simulink model "integracion_control_trayectoria"  (R2023b)
settings: Solver=FixedStepDiscrete  StartTime=0.0  StopTime=inf  RelTol=1e-3  EnableMultiTasking=on
undefined symbols (not defined in the file): LF
libraries: instrumentseriallib x3, svdutilitieslib x1, dspnetwork x1
settings Model: SimulationMode=accelerator  Creator=gianm  LastModifiedBy=gianm
settings DebuggingCC: ParameterPrecisionLossMsg=none

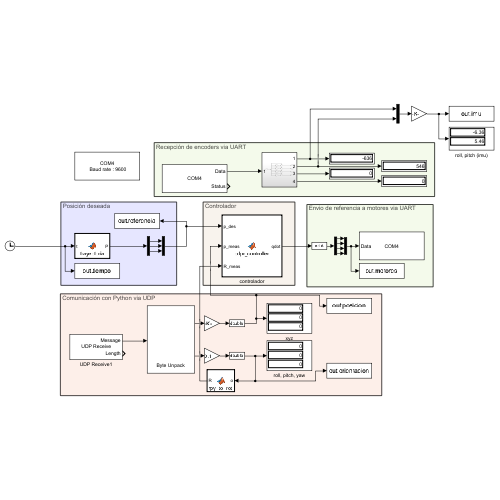
[thumbnail: Simulink's stored preview of the top-level diagram]
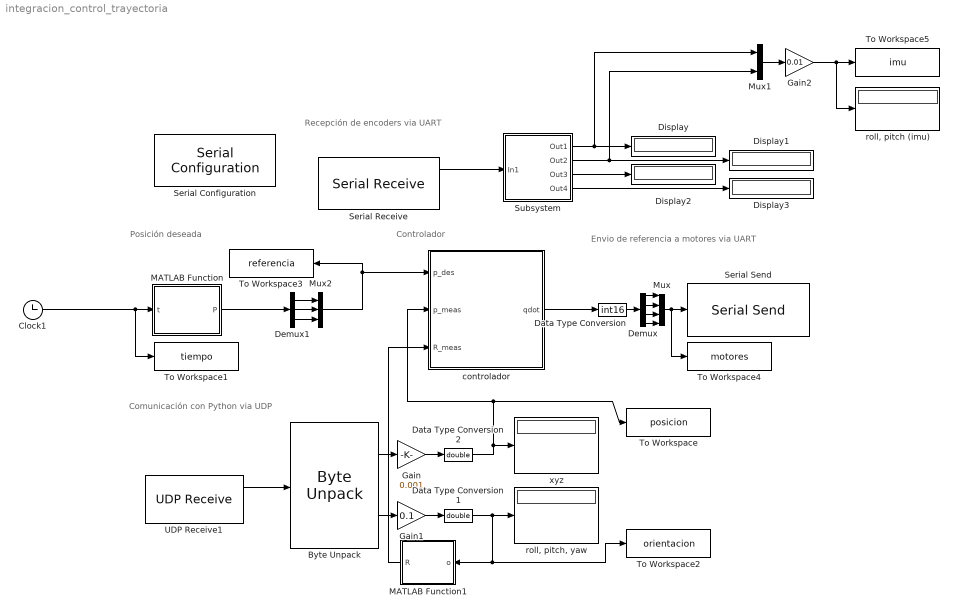
== system integracion_control_trayectoria ==
  note: Recepción de encoders via UART
  note: Controlador
  note: Envio de referencia a motores via UART
  note: Posición deseada
  note: Comunicación con Python via UDP
  Byte Unpack : svdutilitieslib/Byte Unpack  dimensions={[3,1], [3,1]}  datatypes={'int16', 'int16'}  byteAlign=1  blockPlatform=arduinoert
  Clock1 : Clock
  Data Type Conversion : DataTypeConversion  OutDataTypeStr=int16  SaturateOnIntegerOverflow=off  RndMeth=Floor
  Data Type Conversion1 : DataTypeConversion  OutDataTypeStr=double  SaturateOnIntegerOverflow=off  RndMeth=Floor
  Data Type Conversion2 : DataTypeConversion  OutDataTypeStr=double  SaturateOnIntegerOverflow=off  RndMeth=Floor
  Demux : Demux
  Demux1 : Demux  Outputs=3
  Display{,1..3} (4 alike) : Display
      settings: Format=decimal (Stored Integer)
  Gain : Gain  Gain=0.001
  Gain1 : Gain  Gain=0.1
  Gain2 : Gain  Gain=0.01
  MATLAB Function : MATLAB Function  TreatAsAtomicUnit=on
  MATLAB Function1 : MATLAB Function  TreatAsAtomicUnit=on
  Mux : Mux
  Mux1 : Mux  Inputs=2
  Mux2 : Mux  Inputs=3
  Serial Configuration : instrumentseriallib/Serial Configuration  Priority=-200000  PortSel=COM4  Port=COM4  ComPort=COM4  BaudRate=9600  DataBits=8  Parity=none  StopBits=1  ByteOrder=little-endian  FlowControl=none  Timeout=20  SimulateUsing=Interpreted execution  BlockInModel=on  aMode=1
  Serial Receive : instrumentseriallib/Serial Receive  Priority=1  PortSel=COM4  Port=COM4  ComPort=COM4  DataType=uint8  SaveDataType=uint8  ToggleHeader=on  Header=[82]  DataSize=8  ToggleTerminator=on  Terminator=LF ('\n')  CustomTerminator=[]  InputFormat=Column major  ToggleDataSize=on  EnableBlockingMode=off  ActionDataUnavailable=Output last received value  ActionWhenDataUnavailable=Output last received value  CustomValue=0  SampleTime=0.02  SimulateUsing=Interpreted execution  BlockInModel=on  aMode=1
  Serial Send : instrumentseriallib/Serial Send  Priority=1  PortSel=COM4  Port=COM4  ComPort=COM4  Header=[72]  Terminator=LF ('\n')  CustomTerminator=[]  EnableBlockingMode=off  SimulateUsing=Interpreted execution  BlockInModel=on  aMode=1
  Subsystem : Subsystem
  To Workspace : ToWorkspace  VariableName=posicion  SampleTime=0.02
  To Workspace1 : ToWorkspace  VariableName=tiempo  SampleTime=-1
      settings: Save2DSignal=2-D array (concatenate along first dimension)
  To Workspace2 : ToWorkspace  VariableName=orientacion  SampleTime=0.02
  To Workspace3 : ToWorkspace  VariableName=referencia  SampleTime=0.02
      settings: Save2DSignal=2-D array (concatenate along first dimension)
  To Workspace4 : ToWorkspace  VariableName=motores  SampleTime=-1
      settings: Save2DSignal=2-D array (concatenate along first dimension)
  To Workspace5 : ToWorkspace  VariableName=imu  SampleTime=0.02
  UDP Receive1 : dspnetwork/UDP Receive  localURL='0.0.0.0'  localPort=5005  remoteURL='127.0.0.1'  remotePort=-1  recvBufferSize=16  dims=12  signalDatatype=uint8  isComplex=off  isVarSize=off  showBlockingTime=off  blockingTime=0  sampletime=0.02  blockPlatform=[]
      settings: LibrarySourceBlock=dspsrcs4/UDP Receive
  controlador : MATLAB Function  TreatAsAtomicUnit=on
  "roll, pitch (imu)" : Display
  "roll, pitch, yaw" : Display
  xyz : Display
  wires:
  Serial Receive/1 -> Subsystem/1(In1)
  Mux/1 -> Serial Send/1, To Workspace4/1
  Demux/1 -> Mux/1
  Subsystem/1(Out1) -> Display/1, Mux1/1
  Subsystem/4(Out4) -> Display3/1
  Subsystem/3(Out3) -> Display2/1
  Subsystem/2(Out2) -> Display1/1, Mux1/2
  Demux/2 -> Mux/2
  Demux/3 -> Mux/3
  Demux/4 -> Mux/4
  Data Type Conversion/1 -> Demux/1
  Byte Unpack/2 -> Gain1/1
  Byte Unpack/1 -> Gain/1
  UDP Receive1/1 -> Byte Unpack/1
  Mux2/1 -> To Workspace3/1, controlador/1(p_des)
  Data Type Conversion2/1 -> controlador/2(p_meas), To Workspace/1, xyz/1
  Data Type Conversion1/1 -> To Workspace2/1, MATLAB Function1/1(o), "roll, pitch, yaw"/1
  Clock1/1 -> To Workspace1/1, MATLAB Function/1(t)
  Demux1/1 -> Mux2/1
  Demux1/2 -> Mux2/2
  Demux1/3 -> Mux2/3
  MATLAB Function1/1(R) -> controlador/3(R_meas)
  controlador/1(qdot) -> Data Type Conversion/1
  Gain/1 -> Data Type Conversion2/1
  Gain1/1 -> Data Type Conversion1/1
  MATLAB Function/1(P) -> Demux1/1
  Mux1/1 -> Gain2/1
  Gain2/1 -> "roll, pitch (imu)"/1, To Workspace5/1

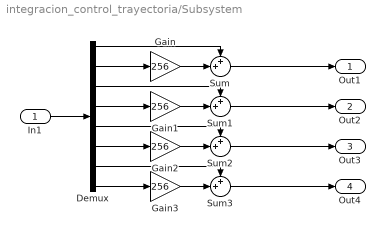
== system integracion_control_trayectoria/Subsystem ==
  In1 : Inport
  Demux : Demux  Outputs=8
  Gain{,1..3} (4 alike) : Gain  Gain=256
  Sum{,1..3} (4 alike) : Sum  Inputs=++|  OutDataTypeStr=int16
  Out1 : Outport
  Out2 : Outport  Port=2
  Out3 : Outport  Port=3
  Out4 : Outport  Port=4
  wires:
  In1/1 -> Demux/1
  Demux/2 -> Gain/1
  Gain/1 -> Sum/2
  Demux/1 -> Sum/1
  Sum/1 -> Out1/1
  Demux/4 -> Gain1/1
  Demux/3 -> Sum1/1
  Gain1/1 -> Sum1/2
  Demux/6 -> Gain2/1
  Sum2/1 -> Out3/1
  Demux/5 -> Sum2/1
  Gain2/1 -> Sum2/2
  Demux/8 -> Gain3/1
  Demux/7 -> Sum3/1
  Gain3/1 -> Sum3/2
  Sum1/1 -> Out2/1
  Sum3/1 -> Out4/1

== matlab function integracion_control_trayectoria/MATLAB Function ==
  data: t input; P output
function P = trayectoria(t)
% ==========================
% DEFINICIÓN DE WAYPOINTS
% ==========================
wp = [
    0    0    0.11
    0    0    0.11
    0    0    0.14
    0    0    0.14
    0.07  0    0.14
    0.07  0    0.14
    0.07  0.07  0.14
    0.07  0.07  0.14
   -0.07  0.07  0.14
   -0.07  0.07  0.14
   -0.07 -0.07  0.14
   -0.07 -0.07  0.14
    0.07 -0.07  0.14
    0.07 -0.07  0.14
    0.07  0    0.14
    0.07  0    0.14
    0    0    0.14
    0    0    0.14
    0    0    0.11
];

% ==========================
% DURACIÓN POR TRAMO
% Debe haber N-1 tiempos
% ==========================

%Tseg = 1*[1 1 1.0 1 1.0 1 1.0 2 1.0 2 1.0 2 1.0 1 1.0 1 1.0 1]; 
Tseg = 2*[2 1 0.5 1 0.5 1 0.5 2 0.5 2 0.5 2 0.5 1 0.5 1 0.5 1];  

%Tseg = 4*[1 1 1 1 2 2 2 1 1 1];   % EJEMPLO... tú colocas lo que quieras

N = size(wp,1) - 1;           % Número de tramos

if length(Tseg) ~= N
    error('El vector Tseg debe tener %d elementos', N);
end

% ==========================
% TIEMPO ACUMULADO POR TRAMO
% ==========================
Tcum = [0, cumsum(Tseg)];

T_total = Tcum(end);


% ==========================
% REPETICIÓN DE LA TRAYECTORIA
% ==========================
% Hace que el tiempo sea cíclico entre 0 y T_total
t = mod(t, T_total);


% ==========================
% CLAMP DE TIEMPO
% ==========================
if t <= 0
    P = wp(1,:);
    return;
elseif t >= T_total
    P = wp(end,:);
    return;
end

% ==========================
% DETERMINAR TRAMO ACTUAL
% ==========================
i = find(t >= Tcum(1:end-1) & t < Tcum(2:end), 1);

% Tiempo local del tramo
t0 = Tcum(i);
t1 = Tcum(i+1);
tau = (t - t0) / (t1 - t0);

% ==========================
% INTERPOLACIÓN LINEAL
% ==========================
p0 = wp(i,:);
p1 = wp(i+1,:);

p_int = p0 + tau * (p1 - p0);

P = [p_int(1), p_int(2), p_int(3)];
end

== matlab function integracion_control_trayectoria/controlador ==
  data: p_des input; qdot output; p_meas input; R_meas input
function qdot = cdpr_controller(p_des, p_meas, R_meas)

% p_des: [3x1] posición deseada
% p_meas: [3x1] posición medida
% R_meas: [3x3] orientación medida
% Output:
%   qdot = velocidades de motores [deg/s]


% anchors: [3x4] posiciones de los anclajes
% offsets: [3x4] offsets desde COM hasta uniones del efector
% Rcarrete: radio del carrete (m/ rad)

% Anclajes de la base (4 esquinas)
anchors = [ 0.27/2  0.27/2 -0.27/2  -0.27/2;
           -0.27/2  0.27/2  0.27/2  -0.27/2;
            0.22    0.22    0.22     0.22]; % (3x4)

% Offsets desde el centro del efector hasta cada esquina
% prisma de 0.1 x 0.1 x 0.030
Lx = 0.1; Ly = 0.1; Lz = 0.0;
offsets = [  Lx  Lx  -Lx  -Lx;
            -Ly  Ly   Ly  -Ly;
             Lz  Lz   Lz   Lz ]/2; % (3x4)

Rcarrete = 0.03/2;

% Kp: ganancia proporcional (0.5 - 2 recomendado)
Kp = 0.5;

%% 1. Error y velocidad deseada
e = p_des - p_meas;

% velocidad deseada del efector
v = Kp * e;

% no controlar orientación → omega = 0
omega = [0;0;0];

%% 2. Construir Jacobiana
J = zeros(4,6);

for i = 1:4
    % posición del punto de unión en global
    Pi = p_meas + R_meas * offsets(:,i);

    % vector del cable
    di = anchors(:,i) - Pi;

    % longitud
    Li = norm(di);

    % dirección del cable
    ui = di / Li;

    % vector desde COM al punto de unión
    ri = R_meas * offsets(:,i);

    % fila de la jacobiana
    J(i,1:3) = -ui';
    J(i,4:6) = (cross(ri, ui))';
end

%% 3. Velocidades de cable
xi = [v; omega];    % 6x1
Ldot = J * xi;      % 4x1

%% 4. Velocidades de motores
qdot = Ldot / Rcarrete;
qdot = qdot * 180 / pi;

qdot = max(min(qdot, 250), -250); % Saturador de velocidad angular

== matlab function integracion_control_trayectoria/MATLAB Function1 ==
  data: o input; R output
function R = rpy_to_rot(o)
% Convierte roll-pitch-yaw (en grados) a matriz de rotación R (3x3)
% Convención: R = Rz(yaw) * Ry(pitch) * Rx(roll)

roll_deg = o(1);
pitch_deg = o(2);
yaw_deg = o(3);

% convertir a radianes
roll  = roll_deg  * pi/180;
pitch = pitch_deg * pi/180;
yaw   = yaw_deg   * pi/180;

% cosenos y senos
cr = cos(roll);  sr = sin(roll);
cp = cos(pitch); sp = sin(pitch);
cy = cos(yaw);   sy = sin(yaw);

% matriz de rotación final
R = zeros(3,3);

R(1,1) = cy*cp;
R(1,2) = cy*sp*sr - sy*cr;
R(1,3) = cy*sp*cr + sy*sr;

R(2,1) = sy*cp;
R(2,2) = sy*sp*sr + cy*cr;
R(2,3) = sy*sp*cr - cy*sr;

R(3,1) = -sp;
R(3,2) = cp*sr;
R(3,3) = cp*cr;
